simulink model "scheme2"  (R2024a)
settings: Solver=VariableStepAuto  StartTime=0.0  StopTime=10.0  RelTol=1e-8
undefined symbols (not defined in the file or in its folder): g, K, T1, T2
settings Model: Creator=alexivanov  LastModifiedBy=alexivanov

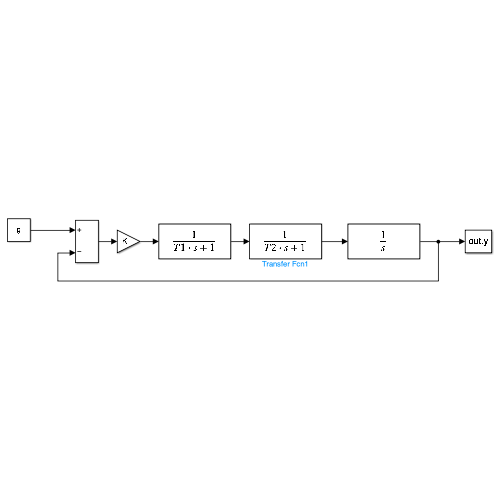
[thumbnail: Simulink's stored preview of the top-level diagram]
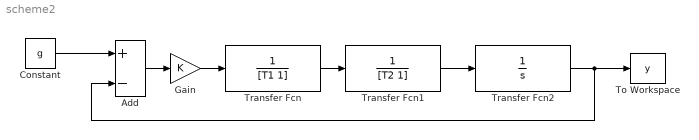
== system scheme2 ==
  Add : Sum  Inputs=+-
  Constant : Constant  Value=g
  Gain : Gain  Gain=K
  To Workspace : ToWorkspace  VariableName=y  SaveFormat=Timeseries  SampleTime=-1
  Transfer Fcn : TransferFcn  Denominator=[T1 1]
  Transfer Fcn1 : TransferFcn  Denominator=[T2 1]
  Transfer Fcn2 : TransferFcn  Denominator=[1, 0]
  wires:
  Constant/1 -> Add/1
  Transfer Fcn/1 -> Transfer Fcn1/1
  Transfer Fcn1/1 -> Transfer Fcn2/1
  Transfer Fcn2/1 -> To Workspace/1, Add/2
  Add/1 -> Gain/1
  Gain/1 -> Transfer Fcn/1
